simulink model "TP1"  (R2023b)
settings: Solver=VariableStepAuto  StartTime=0.0  StopTime=20  RelTol=1e-3
undefined symbols (not defined in the file): A, B, C, E, K, L
settings Model: Creator=robot  LastModifiedBy=robot

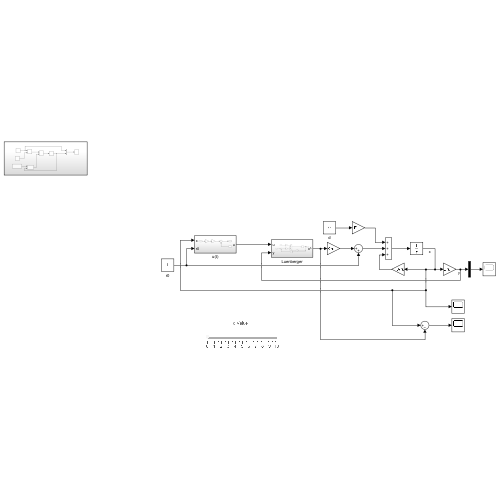
[thumbnail: Simulink's stored preview of the top-level diagram]
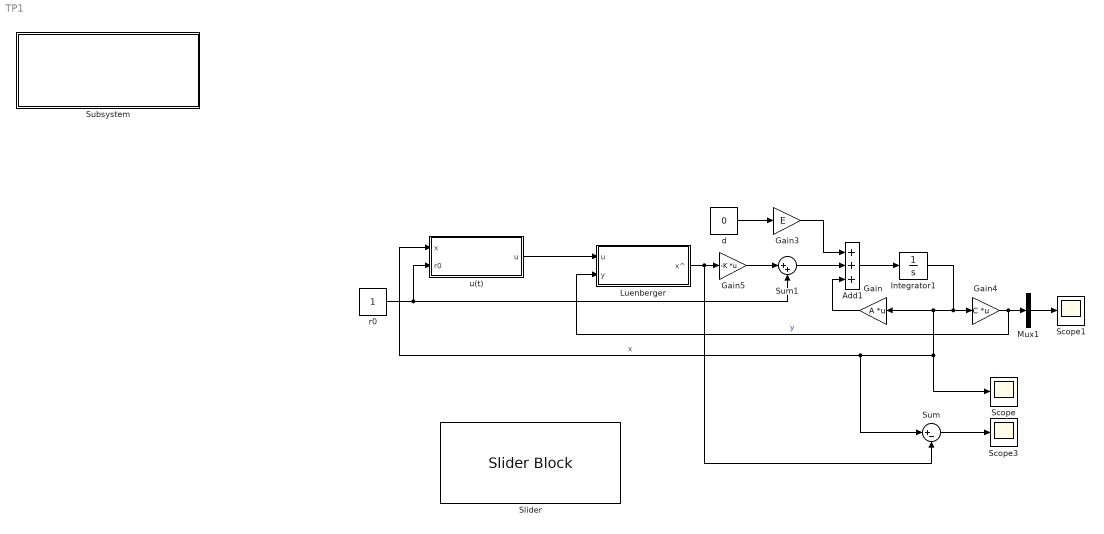
== system TP1 ==
  Add1 : Sum  Inputs=+++
  Gain : Gain  Gain=A  Multiplication=Matrix(K*u)
  Gain3 : Gain  Gain=E
  Gain4 : Gain  Gain=C  Multiplication=Matrix(K*u)
  Gain5 : Gain  Gain=-K  Multiplication=Matrix(K*u)
  Integrator1 : Integrator
  Luenberger : Subsystem
  Mux1 : Mux  Inputs=1
  Scope : Scope
  Scope1 : Scope
  Scope3 : Scope
  Slider : SliderBlock  ScaleMax=10
  Subsystem : Subsystem
  Sum : Sum  Inputs=|+-
  Sum1 : Sum  Inputs=|++
  d : Constant  Value=0
  r0 : Constant
  u(t) : Subsystem
  wires:
  Integrator1/1 -> Scope/1, Sum/1, u(t)/1(x), Gain/1, Gain4/1  "x"
  Add1/1 -> Integrator1/1
  Gain/1 -> Add1/3
  r0/1 -> u(t)/2(r0), Sum1/2
  d/1 -> Gain3/1
  Gain3/1 -> Add1/1
  Mux1/1 -> Scope1/1
  Gain4/1 -> Luenberger/2(y), Mux1/1  "y"
  Luenberger/1(x^) -> Sum/2, Gain5/1
  Gain5/1 -> Sum1/1
  Sum1/1 -> Add1/2
  u(t)/1(u) -> Luenberger/1(u)
  Sum/1 -> Scope3/1

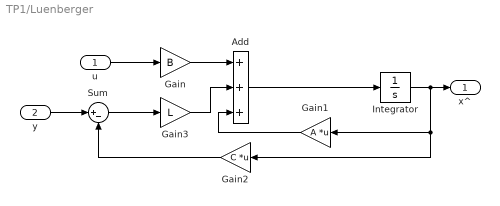
== system TP1/Luenberger ==
  u : Inport
  y : Inport  Port=2
  Add : Sum  Inputs=+++
  Gain : Gain  Gain=B
  Gain1 : Gain  Gain=A  Multiplication=Matrix(K*u)
  Gain2 : Gain  Gain=C  Multiplication=Matrix(K*u)
  Gain3 : Gain  Gain=L
  Integrator : Integrator
  Sum : Sum  Inputs=|+-
  x^ : Outport
  wires:
  y/1 -> Sum/1
  u/1 -> Gain/1
  Sum/1 -> Gain3/1
  Add/1 -> Integrator/1
  Gain/1 -> Add/1
  Gain3/1 -> Add/2
  Gain1/1 -> Add/3
  Gain2/1 -> Sum/2
  Integrator/1 -> Gain2/1, Gain1/1, x^/1

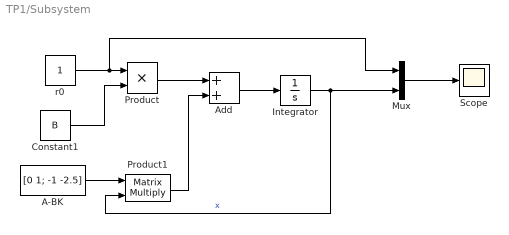
== system TP1/Subsystem ==
  A-BK : Constant  Value=[0 1; -1 -2.5]
  Add : Sum
  Constant1 : Constant  Value=B
  Integrator : Integrator
  Mux : Mux  Inputs=2
  Product : Product
  Product1 : Product  Multiplication=Matrix(*)
  Scope : Scope
  r0 : Constant
  wires:
  Product1/1 -> Add/2
  Constant1/1 -> Product/2
  r0/1 -> Mux/1, Product/1
  Integrator/1 -> Mux/2, Product1/2  "x"
  Mux/1 -> Scope/1
  Product/1 -> Add/1
  A-BK/1 -> Product1/1
  Add/1 -> Integrator/1

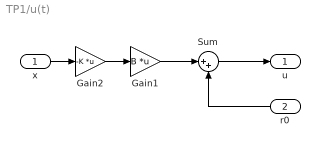
== system TP1/u(t) ==
  x : Inport
  r0 : Inport  Port=2
  Gain1 : Gain  Gain=B  Multiplication=Matrix(K*u)
  Gain2 : Gain  Gain=-K  Multiplication=Matrix(K*u)
  Sum : Sum  Inputs=|++
  u : Outport
  wires:
  x/1 -> Gain2/1
  Gain2/1 -> Gain1/1
  Gain1/1 -> Sum/1
  Sum/1 -> u/1
  r0/1 -> Sum/2
